simulink model "f1"  (R2022a)
settings: Solver=VariableStepAuto  StartTime=0.0  StopTime=10.0  RelTol=1e-3
undefined symbols (not defined in the file): a
settings Model: Creator=Mihai Dinu  LastModifiedBy=Mihai Dinu

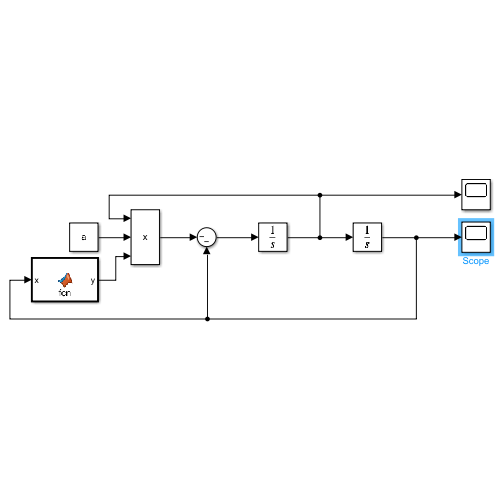
[thumbnail: Simulink's stored preview of the top-level diagram]
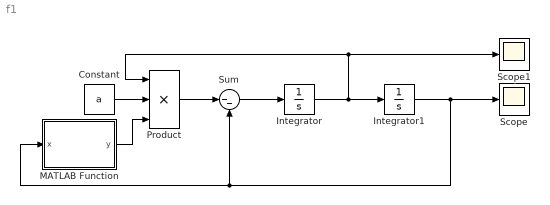
== system f1 ==
  Constant : Constant  Value=a
  Integrator : Integrator  InitialCondition=0.1
  Integrator1 : Integrator  InitialCondition=0.1
  MATLAB Function : MATLAB Function  TreatAsAtomicUnit=on
  Product : Product  Inputs=3
  Scope : Scope
  Scope1 : Scope
  Sum : Sum  Inputs=|--
  wires:
  Integrator/1 -> Integrator1/1, Scope1/1, Product/1
  Integrator1/1 -> MATLAB Function/1(x), Sum/2, Scope/1
  Product/1 -> Sum/1
  Sum/1 -> Integrator/1
  Constant/1 -> Product/2
  MATLAB Function/1(y) -> Product/3

== matlab function f1/MATLAB Function ==
  data: x input; y output
function y = fcn(x)

y = 1-x*x;
